simulink model "PMSM_FOC_sensorless"  (R2026a)
settings: Solver=FixedStepDiscrete  StopTime=10  FixedStep=Ts  EnableMultiTasking=on
InitFcn:
  | ParameterInit
undefined symbols (not defined in the file): drive, FAKF, motor, Ts
libraries: simulink x10, mcbhdlcontrolslib x10, matrix_library x8, mcbcontrolslib x6, mcbpositiondecoderlib x3, mcbsensorlessestimatorlib x2, mcbeeMathTransformLib x2, slpidlib x2, sl_discontinuities x1, mcbplantlib x1, autolibpmsminterior x1, realtime_pacer_lib x1
(part 2 of 3)

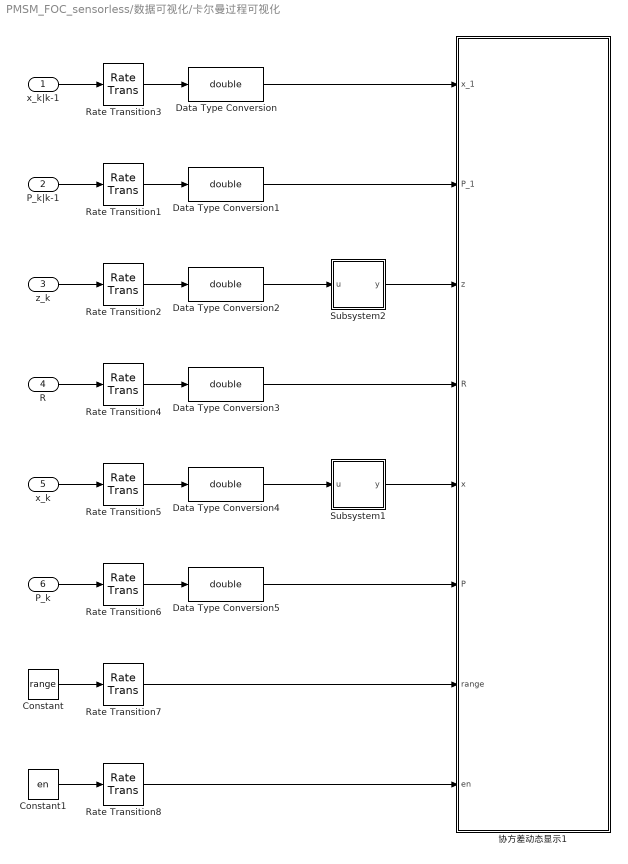
== system PMSM_FOC_sensorless/数据可视化/卡尔曼过程可视化 ==
  x_k|k-1 : Inport
  P_k|k-1 : Inport  Port=2
  z_k : Inport  Port=3
  R : Inport  Port=4
  x_k : Inport  Port=5
  P_k : Inport  Port=6
  Constant : Constant  Value=range
  Constant1 : Constant  Value=en
  Data Type Conversion{,1..5} (6 alike) : DataTypeConversion  OutDataTypeStr=double  SaturateOnIntegerOverflow=off  RndMeth=Floor
  Rate Transition{1..8} (8 alike) : RateTransition  OutPortSampleTime=1/plot_freq
  Subsystem1 : Subsystem
  Subsystem2 : Subsystem
  协方差动态显示1 : MATLAB Function  TreatAsAtomicUnit=on
  wires:
  z_k/1 -> Rate Transition2/1
  x_k/1 -> Rate Transition5/1
  R/1 -> Rate Transition4/1
  Rate Transition2/1 -> Data Type Conversion2/1
  P_k|k-1/1 -> Rate Transition1/1
  x_k|k-1/1 -> Rate Transition3/1
  Rate Transition5/1 -> Data Type Conversion4/1
  Rate Transition4/1 -> Data Type Conversion3/1
  P_k/1 -> Rate Transition6/1
  Rate Transition1/1 -> Data Type Conversion1/1
  Rate Transition3/1 -> Data Type Conversion/1
  Data Type Conversion4/1 -> Subsystem1/1(u)
  Data Type Conversion2/1 -> Subsystem2/1(u)
  Data Type Conversion/1 -> 协方差动态显示1/1(x_1)
  Data Type Conversion3/1 -> 协方差动态显示1/4(R)
  Subsystem2/1(y) -> 协方差动态显示1/3(z)
  Data Type Conversion1/1 -> 协方差动态显示1/2(P_1)
  Subsystem1/1(y) -> 协方差动态显示1/5(x)
  Data Type Conversion5/1 -> 协方差动态显示1/6(P)
  Constant/1 -> Rate Transition7/1
  Rate Transition6/1 -> Data Type Conversion5/1
  Constant1/1 -> Rate Transition8/1
  Rate Transition7/1 -> 协方差动态显示1/7(range)
  Rate Transition8/1 -> 协方差动态显示1/8(en)

== system PMSM_FOC_sensorless/Encoder&Hall/霍尔传感器/Subsystem ==
  MtrPos : Inport
  Constant6 : Constant  Value=pi/6  OutDataTypeStr=single
  Constant7 : Constant  Value=6  OutDataTypeStr=int16
  Data Type Conversion : DataTypeConversion  OutDataTypeStr=single  SaturateOnIntegerOverflow=off  RndMeth=Floor
  Data Type Conversion1 : DataTypeConversion  OutDataTypeStr=int16  SaturateOnIntegerOverflow=off  RndMeth=Floor
  Gain : Gain  Gain=6/(2*pi)
  Mechanical to Electrical Position : mcbpositiondecoderlib/Mechanical to Electrical Position  PolePairsInputType=Specify via dialog  NrPP=motor.P  selectedRange=Radians  MechOfstInputType=Specify via dialog  mechOffsetIn=0  maxAngleIn=2*pi  InputDataType=single  VariantSelect=floating-point
  Mod : Math  Operator=mod
  Sum : Sum  Inputs=|++
  Phase : Outport
  wires:
  Mod/1 -> Phase/1
  Data Type Conversion1/1 -> Mod/1
  Gain/1 -> Data Type Conversion1/1
  Sum/1 -> Gain/1
  Constant6/1 -> Sum/2
  Constant7/1 -> Mod/2
  Data Type Conversion/1 -> Mechanical to Electrical Position/1  "ElecAngle"
  MtrPos/1 -> Data Type Conversion/1
  Mechanical to Electrical Position/1 -> Sum/1

== system PMSM_FOC_sensorless/FOC/Observer/AKF ==
  u_k : Inport
  z_k : Inport  Port=2
  协方差估计 : Subsystem
  协方差计算 : Subsystem
  状态观测 : Subsystem
  x_k : Outport
  tag scope: K=global, Q=global, R=global, S=global, T=global
  wires:
  协方差估计/1(R) -> 协方差计算/1(R), [R]  "R"
  u_k/1 -> 状态观测/1(u)
  z_k/1 -> 状态观测/2(z)
  状态观测/1(x^) -> x_k/1  "x^"
  状态观测/3(e^) -> 协方差估计/2(e^)  "e^"
  状态观测/2(e~) -> 协方差估计/1(e~)  "e~"
  协方差计算/2(S) -> [S], 协方差估计/3(S)  "S"
  协方差估计/2(Q) -> [Q], 协方差计算/2(Q)  "Q"
  协方差计算/1(K) -> [K], 状态观测/3(K)  "K"
  协方差计算/3(T) -> [T], 协方差估计/4(T)  "T"

== system PMSM_FOC_sensorless/FOC/Observer/位置提取 ==
  Eαβ : Inport
  θ_sincos : Inport  Port=2
  Constant : Constant  Value=motor.psi  OutDataTypeStr=single
  Demux : Demux  Outputs=2
  Divide3 : Product  Inputs=/*
  Gain : Gain  Gain=[-1 1]  Multiplication=Matrix(K*u)
  Gain1 : Gain  Gain=motor.P
  Gain2 : Gain  Gain=-1
  Mux : Mux  Inputs=2
  Product : Product
  Product1 : Product
  Sign : Signum
  Unit Delay : UnitDelay  SampleTime=-1
  幅角 : mcbcontrolslib/atan2  ApproximationMethod=None  NumberOfIterations=11  NumberOfDataPoints=16  InterpMethod=Flat  outputUnit=Radians  TableDataTypeStr=Inherit: Inherit via input
  ωθ : Outport
  wires:
  Constant/1 -> Gain1/1
  Gain1/1 -> Divide3/1
  幅角/1 -> Mux/2
  θ_sincos/1 -> Unit Delay/1
  Unit Delay/1 -> Product/1
  Product/1 -> Gain/1
  Gain/1 -> Divide3/2, Sign/1
  Divide3/1 -> Mux/1
  Mux/1 -> ωθ/1
  Demux/2 -> 幅角/2
  Demux/1 -> Gain2/1
  Gain2/1 -> 幅角/1
  Eαβ/1 -> Product/2, Product1/2
  Sign/1 -> Product1/1
  Product1/1 -> Demux/1

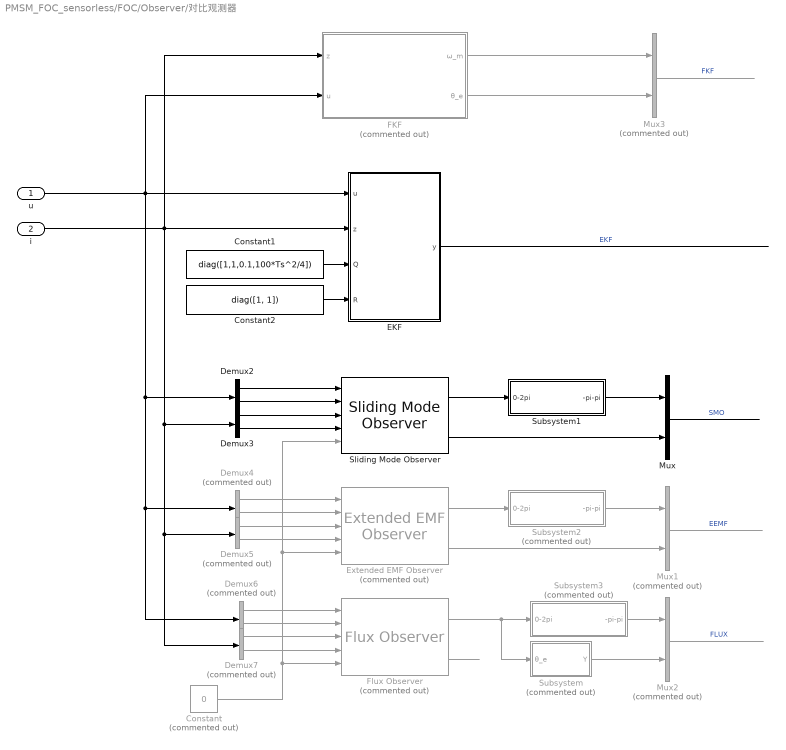
== system PMSM_FOC_sensorless/FOC/Observer/对比观测器 ==
  u : Inport
  i : Inport  Port=2
  Constant : Constant  Commented=on  Value=0  OutDataTypeStr=single
  Constant1 : Constant  Value=diag([1,1,0.1,100*Ts^2/4])  OutDataTypeStr=single
  Constant2 : Constant  Value=diag([1, 1])  OutDataTypeStr=single
  Demux2 : Demux  Outputs=2
  Demux3 : Demux  Outputs=2
  Demux{4..7} (4 alike) : Demux  Commented=on  Outputs=2
  EKF : Subsystem
  Extended EMF Observer : mcbsensorlessestimatorlib/Extended EMF Observer  Commented=on  InputUnit=SI unit  PosOut=Electrical position  BlkSampleTime=Ts  StatorResistance=motor.Rs  StatorDaxisInductance=motor.Ls  StatorQaxisInductance=motor.Ls  MaxApplicationSpeed=3000  PolePairs=motor.P  MaxStatorVoltage=12*sqrt(3)  MaxStatorCurrent=10  Alpha=50  EEMFCutoffFreq=50  Kp=250  Ki=200000  N_points=1024  SpeedCutoffFreq=50  PositionUnit=Radians  PositionDataType=single  SpeedUnit=Radians/sec  PerUnitSpeed=6000  SpeedDataType=single  TableDatatype=single
      settings: LibrarySourceBlock=mcblib/Sensorless Estimators/Extended EMF Observer
  FKF : Subsystem  Commented=on
  Flux Observer : mcbpositiondecoderlib/Flux Observer  Commented=on  MotorSelection=PMSM  DataTypeSelect=off  BlockInputUnit=Per-unit  PerUnitVoltage=12*sqrt(3)  PerUnitCurrent=10  PositionSelect=on  FluxSelect=off  TorqueSelect=on  PolePairs=4  StatorResistance=0.36  StatorDAxisInductance=0.2e-3  StatorLeakageInductance=0.0068  RotorLeakageInductance=0.0068  MagnetizingInductance=0.0300  CutoffFreq=50  BlockSampleTime=Ts  ParameterBusInput=off  PositionUnit=Radians  PositionDatatype=single  FluxUnit=Weber  PerUnitFlux=0.1  FluxDatatype=single  TorqueUnit=Nm  PerUnitTorque=100  TorqueDatatype=single  DataType=0
      settings: LibrarySourceBlock=mcblib/Sensorless Estimators/Flux Observer
  Mux : Mux  Inputs=2
  Mux1 : Mux  Commented=on  Inputs=2
  Mux2 : Mux  Commented=on  Inputs=2
  Mux3 : Mux  Commented=on  Inputs=2
  Sliding Mode Observer : mcbsensorlessestimatorlib/Sliding Mode Observer  InputUnit=Per-unit  BlkSampleTime=Ts  StatorResistance=motor.Rs  StatorInductance=motor.Ls  MaxApplicationSpeed=3000  PolePairs=motor.P  MaxStatorVoltage=12*sqrt(3)  MaxStatorCurrent=10  DisturbanceObserverGain=0.9  CurrentObserverGain=0.5  CutoffFreq=600  PositionUnit=Radians  PositionDataType=single  SpeedUnit=Radians/sec  PerUnitSpeed=6000  SpeedDataType=single
      settings: LibrarySourceBlock=mcblib/Sensorless Estimators/Sliding Mode Observer
  Subsystem : Subsystem  Commented=on
  Subsystem1 : Subsystem
  Subsystem2 : Subsystem  Commented=on
  Subsystem3 : Subsystem  Commented=on
  wires:
  Demux3/2 -> Sliding Mode Observer/4
  Demux2/2 -> Sliding Mode Observer/2
  Demux2/1 -> Sliding Mode Observer/1
  Flux Observer/2 -> ?
  Sliding Mode Observer/2 -> Mux/2
  Demux3/1 -> Sliding Mode Observer/3
  Demux6/2 -> Flux Observer/2
  Demux7/1 -> Flux Observer/3
  Demux6/1 -> Flux Observer/1
  Demux7/2 -> Flux Observer/4
  Constant/1 -> Flux Observer/5, Extended EMF Observer/5, Sliding Mode Observer/5
  Flux Observer/1 -> Subsystem/1(θ_e), Subsystem3/1(0-2pi)
  Extended EMF Observer/1 -> Subsystem2/1(0-2pi)
  Sliding Mode Observer/1 -> Subsystem1/1(0-2pi)
  Extended EMF Observer/2 -> Mux1/2
  Demux5/2 -> Extended EMF Observer/4
  Demux5/1 -> Extended EMF Observer/3
  Demux4/1 -> Extended EMF Observer/1
  Demux4/2 -> Extended EMF Observer/2
  u/1 -> EKF/1(u), FKF/2(u), Demux2/1, Demux4/1, Demux6/1
  Constant2/1 -> EKF/4(R)
  Constant1/1 -> EKF/3(Q)
  i/1 -> Demux3/1, Demux5/1, Demux7/1, FKF/1(z), EKF/2(z)
  EKF/1(y) -> ?  "EKF"
  Subsystem/1(Y) -> Mux2/2
  Mux/1 -> ?  "SMO"
  Mux1/1 -> ?  "EEMF"
  Mux2/1 -> ?  "FLUX"
  FKF/1(ω_m) -> Mux3/1
  FKF/2(θ_e) -> Mux3/2
  Mux3/1 -> ?  "FKF"
  Subsystem1/1(-pi-pi) -> Mux/1
  Subsystem2/1(-pi-pi) -> Mux1/1
  Subsystem3/1(-pi-pi) -> Mux2/1

== system PMSM_FOC_sensorless/FOC/Observer/角度转换 ==
  θ : Inport
  Mux1 : Mux  Inputs=2
  SinCos : Trigonometry  Operator=sincos
  sincos : Outport
  wires:
  SinCos/1 -> Mux1/1
  θ/1 -> SinCos/1
  SinCos/2 -> Mux1/2
  Mux1/1 -> sincos/1

== system PMSM_FOC_sensorless/FOC/Observer/计算转子反电动势 ==
  Iαβ : Inport
  Uαβ : Inport  Port=2
  Sum5 : Sum  Inputs=+--
  滞后补偿 : DiscreteFilter  Numerator=[0 0 1 1]  Denominator=[2 0 0 0]
  电感分压 : simulink/Discrete/Discrete Derivative  gainval=motor.Ls  ICPrevScaledInput=0.0  OutMin=[]  OutMax=[]  OutDataType=fixdt(1, 16)  OutScaling=2^-10  DoSatur=off
  电阻分压 : Gain  Gain=motor.Rs
  Eαβ : Outport
  tag scope: E_alphabeta=global
  wires:
  电感分压/1 -> Sum5/3
  电阻分压/1 -> Sum5/2
  Uαβ/1 -> 滞后补偿/1
  Iαβ/1 -> 电感分压/1, 电阻分压/1
  滞后补偿/1 -> Sum5/1
  Sum5/1 -> Eαβ/1, [E_alphabeta]

== system PMSM_FOC_sensorless/FOC/Observer/转矩计算 ==
  θ_sincos : Inport
  I_αβ : Inport  Port=2
  Constant : Constant  Value=motor.psi  OutDataTypeStr=single
  Divide1 : Product  Inputs=**
  Gain : Gain  Gain=[-1 1]  Multiplication=Matrix(K*u)
  Gain1 : Gain  Gain=motor.P
  Gain2 : Gain  Gain=1.5
  Product3 : Product
  Unit Delay : UnitDelay  SampleTime=-1
  T : Outport
  wires:
  Product3/1 -> Gain/1
  Constant/1 -> Gain1/1
  Divide1/1 -> Gain2/1
  Gain/1 -> Divide1/1
  Unit Delay/1 -> Product3/1
  I_αβ/1 -> Product3/2
  θ_sincos/1 -> Unit Delay/1
  Gain1/1 -> Divide1/2
  Gain2/1 -> T/1

== system PMSM_FOC_sensorless/FOC/PWM调制&故障诊断/故障诊断 ==
  note: 过流保护
  note: 故障码位数说明（暂定）
      |
      | 位
      | 15
      | 14
      | 13
      | 12
      | 11
      | 10
      | 9
      | 8
      | 7
      | 6
      | 5
      | 4
      | 3
      | 2
      | 1
      | 0
      |
      | 说明
      | -
      | -
      | -
      | -
      | -
      | -
      | -
      | -
      | -
      | -
      | -
      | -
      | 过热
      | 过压
      | 欠压
      | 过流
      |
      | 位
      | 31
      | 30
      | 29
      | 28
      | 27
      | 26
      | 25
      | 24
      | 23
      | 22
      | 21
      | 20
      | 19
      | 18
      | 17
      | 16
      |
      | 说明
      | ​
      | ​
      | ​
      | ​
      | ​
      | ​
      | ​
      | ​
      | ​
      | ​
      | ​
      | ​
      | ​
      | ​
      | ​
      | ​
  note: 欠压过压保护
  I_abc : Inport
  U_bus : Inport  Port=2
  Abs : Abs  SaturateOnIntegerOverflow=off
  Bitwise Operator1 : simulink/Logic and Bit Operations/Bitwise Operator  logicop=OR  UseBitMask=off  NumInputPorts=3  BitMask=bin2dec('11011001')  BitMaskRealWorld=Stored Integer
  Constant1 : Constant  Value=drive.V_min
  Constant2 : Constant  Value=drive.I_max
  Constant3 : Constant  Value=drive.V_max
  Gain1 : Gain  Gain=0x2  OutDataTypeStr=uint32
  Gain2 : Gain  Gain=0x4  OutDataTypeStr=uint32
  Gain4 : Gain  Gain=0x1  OutDataTypeStr=uint32
  IIR Filter : mcbhdlcontrolslib/IIR Filter  VariantControl=Low Pass Filter  VariantSelect=Low-pass  FilterConstantInputType=Specify via dialog  Filter_constant=0.1  advancedSettings=off  Ts=50e-6  cutOff_freq=353.6777
  Max : MinMax  Function=max
  OR : Logic  Operator=OR  IconShape=distinctive  AllPortsSameDT=off  OutDataTypeStr=boolean
  Relational Operator : RelationalOperator  Operator=>  OutDataTypeStr=boolean  RndMeth=Simplest  InputSameDT=off
  Relational Operator1 : RelationalOperator  Operator=>  OutDataTypeStr=boolean  RndMeth=Simplest  InputSameDT=off
  Relational Operator2 : RelationalOperator  Operator=<  OutDataTypeStr=boolean  RndMeth=Simplest  InputSameDT=off
  Unit Delay : UnitDelay  SampleTime=-1
  Err_code : Outport
  tag scope: Err_code=global
  wires:
  U_bus/1 -> Relational Operator1/1, Relational Operator2/1
  I_abc/1 -> IIR Filter/1
  Abs/1 -> Max/1
  Constant2/1 -> Relational Operator/2
  Constant1/1 -> Relational Operator2/2
  Relational Operator2/1 -> Gain1/1
  Max/1 -> Relational Operator/1
  Relational Operator1/1 -> Gain2/1
  Constant3/1 -> Relational Operator1/2
  Unit Delay/1 -> OR/1
  Bitwise Operator1/1 -> [Err_code], Err_code/1
  IIR Filter/1 -> Abs/1
  Relational Operator/1 -> OR/2
  Gain2/1 -> Bitwise Operator1/3
  Gain1/1 -> Bitwise Operator1/2
  Gain4/1 -> Bitwise Operator1/1
  OR/1 -> Unit Delay/1, Gain4/1

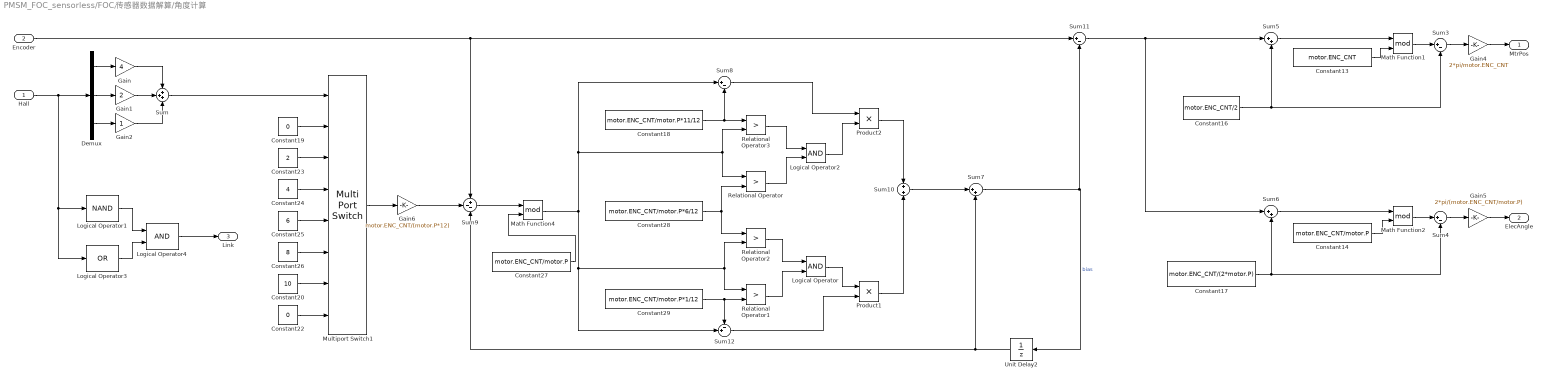
== system PMSM_FOC_sensorless/FOC/传感器数据解算/角度计算 ==
  Hall : Inport
  Encoder : Inport  Port=2
  Constant13 : Constant  Value=motor.ENC_CNT  OutDataTypeStr=int16
  Constant14 : Constant  Value=motor.ENC_CNT/motor.P  OutDataTypeStr=int16
  Constant16 : Constant  Value=motor.ENC_CNT/2  OutDataTypeStr=int16
  Constant17 : Constant  Value=motor.ENC_CNT/(2*motor.P)  OutDataTypeStr=int16
  Constant18 : Constant  Value=motor.ENC_CNT/motor.P*11/12  OutDataTypeStr=int16
  Constant19 : Constant  Value=0  OutDataTypeStr=int16
  Constant20 : Constant  Value=10  OutDataTypeStr=int16
  Constant22 : Constant  Value=0  OutDataTypeStr=int16
  Constant23 : Constant  Value=2  OutDataTypeStr=int16
  Constant24 : Constant  Value=4  OutDataTypeStr=int16
  Constant25 : Constant  Value=6  OutDataTypeStr=int16
  Constant26 : Constant  Value=8  OutDataTypeStr=int16
  Constant27 : Constant  Value=motor.ENC_CNT/motor.P  OutDataTypeStr=int16
  Constant28 : Constant  Value=motor.ENC_CNT/motor.P*6/12  OutDataTypeStr=int16
  Constant29 : Constant  Value=motor.ENC_CNT/motor.P*1/12  OutDataTypeStr=int16
  Demux : Demux  Outputs=3
  Gain : Gain  Gain=4
  Gain1 : Gain  Gain=2
  Gain2 : Gain
  Gain4 : Gain  Gain=2*pi/motor.ENC_CNT  OutDataTypeStr=single
  Gain5 : Gain  Gain=2*pi/(motor.ENC_CNT/motor.P)  OutDataTypeStr=single
  Gain6 : Gain  Gain=motor.ENC_CNT/(motor.P*12)  OutDataTypeStr=int16
  Logical Operator : Logic  AllPortsSameDT=off  OutDataTypeStr=boolean
  Logical Operator1 : Logic  Operator=NAND  Inputs=1  IconShape=distinctive  AllPortsSameDT=off  OutDataTypeStr=boolean
  Logical Operator2 : Logic  AllPortsSameDT=off  OutDataTypeStr=boolean
  Logical Operator3 : Logic  Operator=OR  Inputs=1  IconShape=distinctive  AllPortsSameDT=off  OutDataTypeStr=boolean
  Logical Operator4 : Logic  IconShape=distinctive  AllPortsSameDT=off  OutDataTypeStr=boolean
  Math Function1 : Math  Operator=mod
  Math Function2 : Math  Operator=mod
  Math Function4 : Math  Operator=mod
  Multiport Switch1 : MultiPortSwitch  DataPortOrder=Specify indices  DataPortIndices={5,4,6,2,3,1}  DataPortForDefault=Additional data port  DiagnosticForDefault=None  SaturateOnIntegerOverflow=off  InputSameDT=off
  Product1 : Product  Inputs=**
  Product2 : Product  Inputs=**
  Relational Operator{,1..3} (4 alike) : RelationalOperator  Operator=>  OutDataTypeStr=boolean  RndMeth=Simplest  InputSameDT=off
  Sum : Sum  Inputs=+++
  Sum10 : Sum  Inputs=+|+
  Sum{3..4,8,11} (4 alike) : Sum  Inputs=|+-
  Sum12 : Sum  Inputs=-+|
  Sum5 : Sum  Inputs=|++
  Sum6 : Sum  Inputs=|++
  Sum7 : Sum  Inputs=|++
  Sum9 : Sum  Inputs=+--
  Unit Delay2 : UnitDelay  SampleTime=-1
  MtrPos : Outport
  ElecAngle : Outport  Port=2
  Link : Outport  Port=3
  wires:
  Sum6/1 -> Math Function2/1
  Sum5/1 -> Math Function1/1
  Constant17/1 -> Sum6/2, Sum4/2
  Constant16/1 -> Sum3/2, Sum5/2
  Math Function2/1 -> Sum4/1
  Math Function1/1 -> Sum3/1
  Gain5/1 -> ElecAngle/1
  Gain4/1 -> MtrPos/1
  Sum3/1 -> Gain4/1
  Constant14/1 -> Math Function2/2
  Sum11/1 -> Sum6/1, Sum5/1
  Constant13/1 -> Math Function1/2
  Sum4/1 -> Gain5/1
  Demux/1 -> Gain/1
  Hall/1 -> Demux/1, Logical Operator3/1, Logical Operator1/1
  Gain/1 -> Sum/1
  Demux/2 -> Gain1/1
  Demux/3 -> Gain2/1
  Gain1/1 -> Sum/2
  Gain2/1 -> Sum/3
  Logical Operator4/1 -> Link/1
  Logical Operator1/1 -> Logical Operator4/1
  Logical Operator3/1 -> Logical Operator4/2
  Constant26/1 -> Multiport Switch1/6
  Constant24/1 -> Multiport Switch1/4
  Constant25/1 -> Multiport Switch1/5
  Constant20/1 -> Multiport Switch1/7
  Relational Operator2/1 -> Logical Operator/1
  Constant28/1 -> Relational Operator/2, Relational Operator2/1
  Constant27/1 -> Math Function4/2
  Relational Operator/1 -> Logical Operator2/2
  Constant19/1 -> Multiport Switch1/2
  Unit Delay2/1 -> Sum7/2, Sum9/3
  Sum9/1 -> Math Function4/1
  Constant22/1 -> Multiport Switch1/8
  Logical Operator/1 -> Product1/1
  Multiport Switch1/1 -> Gain6/1
  Constant29/1 -> Sum12/1, Relational Operator1/2
  Product1/1 -> Sum10/2
  Relational Operator3/1 -> Logical Operator2/1
  Constant18/1 -> Sum8/2, Relational Operator3/1
  Sum8/1 -> Product2/1
  Math Function4/1 -> Sum8/1, Relational Operator/1, Relational Operator3/2, Sum12/2, Relational Operator2/2, Relational Operator1/1
  Gain6/1 -> Sum9/2
  Sum12/1 -> Product1/2
  Constant23/1 -> Multiport Switch1/3
  Sum7/1 -> Unit Delay2/1, Sum11/2  "bias"
  Relational Operator1/1 -> Logical Operator/2
  Encoder/1 -> Sum9/1, Sum11/1
  Logical Operator2/1 -> Product2/2
  Product2/1 -> Sum10/1
  Sum10/1 -> Sum7/1
  Sum/1 -> Multiport Switch1/1

== system PMSM_FOC_sensorless/FOC/传感器数据解算/转速计算 ==
  note: 五阶巴特沃斯滤波器
  Encoder : Inport
  Constant3 : Constant  Value=motor.ENC_CNT/2  OutDataTypeStr=int16
  Constant4 : Constant  Value=-motor.ENC_CNT/2  OutDataTypeStr=int16
  Difference : simulink/Discrete/Difference  ICPrevInput=0.0  OutMin=[]  OutMax=[]  OutDataType=fixdt(1, 16)  OutScaling=2^-10  DoSatur=off
  Gain : Gain  Gain=2*pi/motor.ENC_CNT  OutDataTypeStr=single
  Gain1 : Gain  Gain=-motor.ENC_CNT  OutDataTypeStr=int16
  Gain2 : Gain  Gain=motor.ENC_CNT  OutDataTypeStr=int16
  Gain3 : Gain  Gain=1/Ts  OutDataTypeStr=single
  IIR Filter{,1..4} (5 alike) : mcbhdlcontrolslib/IIR Filter  VariantControl=Low Pass Filter  VariantSelect=Low-pass  FilterConstantInputType=Specify via dialog  Filter_constant=0.5  advancedSettings=off  Ts=50e-6  cutOff_freq=3183.0989
  Relational Operator : RelationalOperator  Operator=<  RndMeth=Simplest  InputSameDT=off
  Relational Operator1 : RelationalOperator  Operator=<  RndMeth=Simplest  InputSameDT=off
  Sum2 : Sum  Inputs=+++
  MtrSpeed : Outport
  wires:
  Difference/1 -> Relational Operator1/2, Relational Operator/1, Sum2/2
  Gain2/1 -> Sum2/3
  Gain/1 -> IIR Filter/1
  Constant3/1 -> Relational Operator1/1
  Gain3/1 -> Gain/1
  Gain1/1 -> Sum2/1
  Constant4/1 -> Relational Operator/2
  Relational Operator1/1 -> Gain1/1
  Encoder/1 -> Difference/1
  Relational Operator/1 -> Gain2/1
  IIR Filter/1 -> IIR Filter1/1
  IIR Filter1/1 -> IIR Filter2/1
  Sum2/1 -> Gain3/1
  IIR Filter2/1 -> IIR Filter3/1
  IIR Filter3/1 -> IIR Filter4/1
  IIR Filter4/1 -> MtrSpeed/1

== system PMSM_FOC_sensorless/FOC/全速域电流分配/MJPA ==
  note: $J\left( u_{bus},\omega _m,i_d \right) =-L\frac{{\omega _{mc}}^2}{{\omega _{mc}}^2+{\omega _m}^2}i_d+{Mi_d}^2+\frac{N}{{u_{bus}}^2/3-p_n\omega _m\left( \psi _f+L_di_d \right) ^2}$
  Vbus : Inport
  ω_m : Inport  Port=2
  IIR Filter : mcbhdlcontrolslib/IIR Filter  VariantControl=Low Pass Filter  VariantSelect=Low-pass  FilterConstantInputType=Specify via dialog  Filter_constant=0.1  advancedSettings=off  Ts=50e-6  cutOff_freq=353.6777
  J_function1 : Subsystem  ReferencedSubsystem=J_function
  J_function2 : Subsystem  Commented=on  ReferencedSubsystem=J_function
  J_function3 : Subsystem  ReferencedSubsystem=J_function
  Saturation1 : Saturate  UpperLimit=0.1  LowerLimit=-0.1
  Saturation2 : Saturate  UpperLimit=min(motor.I_rated*1.2)  LowerLimit=max(-motor.I_rated*1.2, -motor.psi/motor.Ls)
  Subsystem2 : Subsystem  Commented=on
  Sum2 : Sum  Inputs=|++
  Sum3 : Sum  Inputs=+|-
  Sum4 : Sum  Inputs=|-+
  Unit Delay : UnitDelay  SampleTime=-1
  Δid : Constant  Value=1e-2  OutDataTypeStr=single
  收敛系数 : Gain  Gain=100
  i*_d : Outport
  wires:
  Saturation1/1 -> Sum4/1
  Δid/1 -> Sum2/1
  Sum2/1 -> J_function1/1
  J_function1/1 -> Sum3/1
  Sum3/1 -> 收敛系数/1  "ΔJ"
  Unit Delay/1 -> Sum4/2, Sum2/2, J_function3/1
  J_function3/1 -> Sum3/2
  Vbus/1 -> J_function3/3, J_function1/3
  收敛系数/1 -> Saturation1/1
  ω_m/1 -> J_function3/2, J_function1/2
  Sum4/1 -> Saturation2/1  "i_d"
  Saturation2/1 -> IIR Filter/1, Unit Delay/1
  IIR Filter/1 -> i*_d/1

== system PMSM_FOC_sensorless/FOC/坐标变换/Subsystem11 ==
  angle : Inport
  Mux : Mux  Inputs=2
  SinCos : Trigonometry  Operator=sincos
  sincos : Outport
  wires:
  SinCos/1 -> Mux/1
  Mux/1 -> sincos/1
  SinCos/2 -> Mux/2
  angle/1 -> SinCos/1

== system PMSM_FOC_sensorless/FOC/坐标变换/Subsystem2 ==
  αβ : Inport
  sincos : Inport  Port=2
  Demux : Demux  Outputs=2
  Demux1 : Demux  Outputs=2
  Mux : Mux  Inputs=2
  Park Transform : mcbeeMathTransformLib/Clarke to Park Angle Transform  AxisAlignment=D-axis  UseWithEmbedded=on  PhaseInput=Two inputs  ThetaInput=Sine and Cosine electrical position  AngleInput=Per-unit  N_points=1024
  dq : Outport
  wires:
  sincos/1 -> Demux1/1
  Demux/2 -> Park Transform/2
  Mux/1 -> dq/1
  Demux/1 -> Park Transform/1
  Demux1/1 -> Park Transform/3
  αβ/1 -> Demux/1
  Demux1/2 -> Park Transform/4
  Park Transform/1 -> Mux/1
  Park Transform/2 -> Mux/2

== system PMSM_FOC_sensorless/FOC/坐标变换/Subsystem3 ==
  abc : Inport
  Gain : Gain  Gain=[2/3 -1/3 -1/3;0 sqrt(3)/3 -sqrt(3)/3]  Multiplication=Matrix(K*u)
  αβ : Outport
  wires:
  abc/1 -> Gain/1
  Gain/1 -> αβ/1

== system PMSM_FOC_sensorless/FOC/坐标变换/Subsystem4 ==
  αβ : Inport
  Demux1 : Demux  Outputs=2
  Gain : Gain  Gain=sqrt(3)/2
  Mux1 : Mux  Inputs=3
  PWM Reference Generator : mcbcontrolslib/PWM Reference Generator  modType=SVM: space vector modulation  inSignal=Valphabeta  expandVoltageInput=on  inputUnits=Per-unit  LimitModulation=off  enableVoltage=on  enableModulationSignal=off  enableDutyCycle=off  expandVoltageOutput=on
  abc : Outport
  wires:
  αβ/1 -> Demux1/1
  Mux1/1 -> Gain/1
  Demux1/1 -> PWM Reference Generator/1
  Demux1/2 -> PWM Reference Generator/2
  PWM Reference Generator/3 -> Mux1/3
  PWM Reference Generator/1 -> Mux1/1
  PWM Reference Generator/2 -> Mux1/2
  Gain/1 -> abc/1

== system PMSM_FOC_sensorless/FOC/坐标变换/Subsystem5 ==
  dq : Inport
  sincos : Inport  Port=2
  Demux : Demux  Outputs=2
  Demux1 : Demux  Outputs=2
  Inverse Park Transform : mcbeeMathTransformLib/Park to Clarke Angle Transform  AxisAlignment=D-axis  UseWithEmbedded=on  PhaseInput=Two inputs  ThetaInput=Sine and Cosine electrical position  AngleInput=Per-unit  N_points=1024
  Mux : Mux  Inputs=2
  αβ : Outport
  wires:
  sincos/1 -> Demux1/1
  Demux1/1 -> Inverse Park Transform/3
  Demux/1 -> Inverse Park Transform/1
  dq/1 -> Demux/1
  Demux/2 -> Inverse Park Transform/2
  Inverse Park Transform/1 -> Mux/1
  Inverse Park Transform/2 -> Mux/2
  Mux/1 -> αβ/1
  Demux1/2 -> Inverse Park Transform/4

== system PMSM_FOC_sensorless/FOC/电流控制/前馈控制1 ==
  ω : Inport
  IdqRef : Inport  Port=2
  IdqFb : Inport  Port=3
  Demux : Demux  Outputs=2
  Demux1 : Demux  Outputs=2
  Discrete Derivative : simulink/Discrete/Discrete Derivative  gainval=motor.Ls  ICPrevScaledInput=0.0  OutMin=[]  OutMax=[]  OutDataType=fixdt(1, 16)  OutScaling=2^-10  DoSatur=off
  Discrete Derivative1 : simulink/Discrete/Discrete Derivative  gainval=motor.Ls  ICPrevScaledInput=0.0  OutMin=[]  OutMax=[]  OutDataType=fixdt(1, 16)  OutScaling=2^-10  DoSatur=off
  Divide1 : Product  Inputs=**
  Divide2 : Product  Inputs=**
  Ld : Gain  Gain=motor.P*motor.Ls
  Lq : Gain  Gain=motor.P*motor.Ls
  Mux : Mux  Inputs=2
  R1 : Gain  Gain=motor.Rs
  R2 : Gain  Gain=motor.Rs
  Sum : Sum  Inputs=+++
  Sum3 : Sum  Inputs=|++
  Sum4 : Sum  Inputs=++-
  转子磁链1 : Constant  Value=motor.P*motor.psi  VectorParams1D=off  OutDataTypeStr=single
  FeedForward : Outport
  wires:
  Demux1/1 -> Discrete Derivative/1  "id"
  Mux/1 -> FeedForward/1
  Discrete Derivative/1 -> Sum4/1
  Discrete Derivative1/1 -> Sum/1
  R1/1 -> Sum4/2  "电阻压降"
  R2/1 -> Sum/2  "电阻压降"
  Demux1/2 -> Discrete Derivative1/1  "iq"
  IdqRef/1 -> Demux1/1
  Sum4/1 -> Mux/1
  Sum/1 -> Mux/2
  Divide1/1 -> Sum/3
  Divide2/1 -> Sum4/3
  IdqFb/1 -> Demux/1
  Demux/2 -> R2/1, Lq/1  "iq*"
  Demux/1 -> Ld/1, R1/1  "id*"
  ω/1 -> Divide1/2, Divide2/2
  Sum3/1 -> Divide1/1
  Lq/1 -> Divide2/1  "定子磁链"
  转子磁链1/1 -> Sum3/2
  Ld/1 -> Sum3/1  "定子磁链"

== system PMSM_FOC_sensorless/FOC/电流控制/电压限幅 ==
  dq_in : Inport
  Limit : Inport  Port=2
  Divide1 : Product  Inputs=*/*
  Math Function1 : Math  Operator=square
  Relational Operator : RelationalOperator  Operator=>  OutDataTypeStr=boolean  RndMeth=Simplest  InputSameDT=off
  Sqrt : Sqrt
  Sum of Elements1 : Sum  Inputs=+
  Switch : Switch  Criteria=u2 > Threshold  SaturateOnIntegerOverflow=off  InputSameDT=off
  dq_out : Outport
  wires:
  dq_in/1 -> Math Function1/1, Switch/3, Divide1/3
  Limit/1 -> Divide1/1, Relational Operator/2
  Sqrt/1 -> Divide1/2, Relational Operator/1
  Sum of Elements1/1 -> Sqrt/1
  Switch/1 -> dq_out/1
  Math Function1/1 -> Sum of Elements1/1
  Relational Operator/1 -> Switch/2
  Divide1/1 -> Switch/1

== system PMSM_FOC_sensorless/FOC/电流控制/非线性补偿 ==
  U_dq : Inport
  Gain1 : Gain  Gain=[1/(motor.Rs+motor.Ls/Ts) 1/(motor.Rs+motor.Ls/Ts)]
  I_dq : Outport
  wires:
  Gain1/1 -> I_dq/1
  U_dq/1 -> Gain1/1

== system PMSM_FOC_sensorless/数据可视化/卡尔曼过程可视化/Subsystem1 ==
  u : Inport
  MATLAB Function : MATLAB Function  TreatAsAtomicUnit=on
  Unit Delay : UnitDelay  InitialCondition=zeros(2,buff_len)  SampleTime=-1
  y : Outport
  wires:
  MATLAB Function/1(y) -> y/1, Unit Delay/1
  Unit Delay/1 -> MATLAB Function/2(y_1)
  u/1 -> MATLAB Function/1(u)

== system PMSM_FOC_sensorless/数据可视化/卡尔曼过程可视化/Subsystem2 ==
  u : Inport
  MATLAB Function : MATLAB Function  TreatAsAtomicUnit=on
  Unit Delay : UnitDelay  InitialCondition=zeros(2,buff_len)  SampleTime=-1
  y : Outport
  wires:
  u/1 -> MATLAB Function/1(u)
  Unit Delay/1 -> MATLAB Function/2(y_1)
  MATLAB Function/1(y) -> Unit Delay/1, y/1

== system PMSM_FOC_sensorless/FOC/Observer/AKF/协方差估计 ==
  e~ : Inport
  e^ : Inport  Port=2
  S : Inport  Port=3
  T : Inport  Port=4
  Display : Display
  Display1 : Display
  Unit Delay1 : UnitDelay  InitialCondition=eye(2)  SampleTime=-1
  Unit Delay2 : UnitDelay  InitialCondition=eye(2)  SampleTime=-1
  乘法积分器 : Subsystem
  乘法积分器1 : Subsystem
  息差估计 : Subsystem
  残差估计 : Subsystem
  R : Outport
  Q : Outport  Port=2
  wires:
  e~/1 -> 息差估计/1(ωθ)
  残差估计/1(cov) -> 乘法积分器/1(S~)
  e^/1 -> 残差估计/1(ωθ)
  S/1 -> Unit Delay1/1
  息差估计/1(cov) -> 乘法积分器1/1(T~)
  Unit Delay1/1 -> 乘法积分器/2(S)
  乘法积分器1/1(R) -> Display1/1, R/1
  乘法积分器/1(Q) -> Display/1, Q/1
  T/1 -> Unit Delay2/1
  Unit Delay2/1 -> 乘法积分器1/2(T)

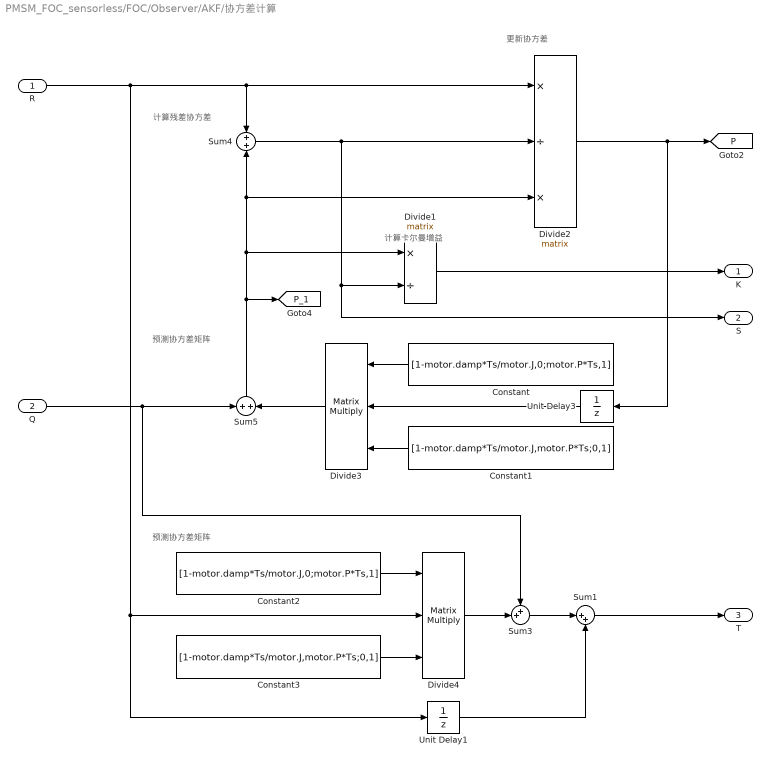
== system PMSM_FOC_sensorless/FOC/Observer/AKF/协方差计算 ==
  note: 预测协方差矩阵
  note: 计算残差协方差
  note: 计算卡尔曼增益
  note: 更新协方差
  note: 预测协方差矩阵
  R : Inport
  Q : Inport  Port=2
  Constant : Constant  Value=[1-motor.damp*Ts/motor.J,0;motor.P*Ts,1]  VectorParams1D=off  OutDataTypeStr=single
  Constant1 : Constant  Value=[1-motor.damp*Ts/motor.J,motor.P*Ts;0,1]  VectorParams1D=off  OutDataTypeStr=single
  Constant2 : Constant  Value=[1-motor.damp*Ts/motor.J,0;motor.P*Ts,1]  VectorParams1D=off  OutDataTypeStr=single
  Constant3 : Constant  Value=[1-motor.damp*Ts/motor.J,motor.P*Ts;0,1]  VectorParams1D=off  OutDataTypeStr=single
  Divide1 : Product  Inputs=*/  Multiplication=Matrix(*)
  Divide2 : Product  Inputs=*/*  Multiplication=Matrix(*)
  Divide3 : Product  Inputs=***  Multiplication=Matrix(*)
  Divide4 : Product  Inputs=***  Multiplication=Matrix(*)
  Sum1 : Sum  Inputs=|++
  Sum3 : Sum  Inputs=++|
  Sum4 : Sum  Inputs=+|+
  Sum5 : Sum  Inputs=+|+
  Unit Delay1 : UnitDelay  InitialCondition=eye(2)  SampleTime=-1
  Unit Delay3 : UnitDelay  InitialCondition=eye(2)  SampleTime=-1
  K : Outport
  S : Outport  Port=2
  T : Outport  Port=3
  tag scope: P=global, P_1=global
  wires:
  Sum5/1 -> [P_1], Divide1/1, Divide2/3, Sum4/2
  Constant/1 -> Divide3/1
  Divide2/1 -> [P], Unit Delay3/1
  Divide3/1 -> Sum5/2
  Constant1/1 -> Divide3/3
  Unit Delay3/1 -> Divide3/2
  Sum4/1 -> S/1, Divide1/2, Divide2/2
  Divide1/1 -> K/1
  Constant3/1 -> Divide4/3
  Constant2/1 -> Divide4/1
  Divide4/1 -> Sum3/2
  Sum3/1 -> Sum1/1
  R/1 -> Unit Delay1/1, Divide4/2, Divide2/1, Sum4/1
  Sum1/1 -> T/1
  Unit Delay1/1 -> Sum1/2
  Q/1 -> Sum3/1, Sum5/1

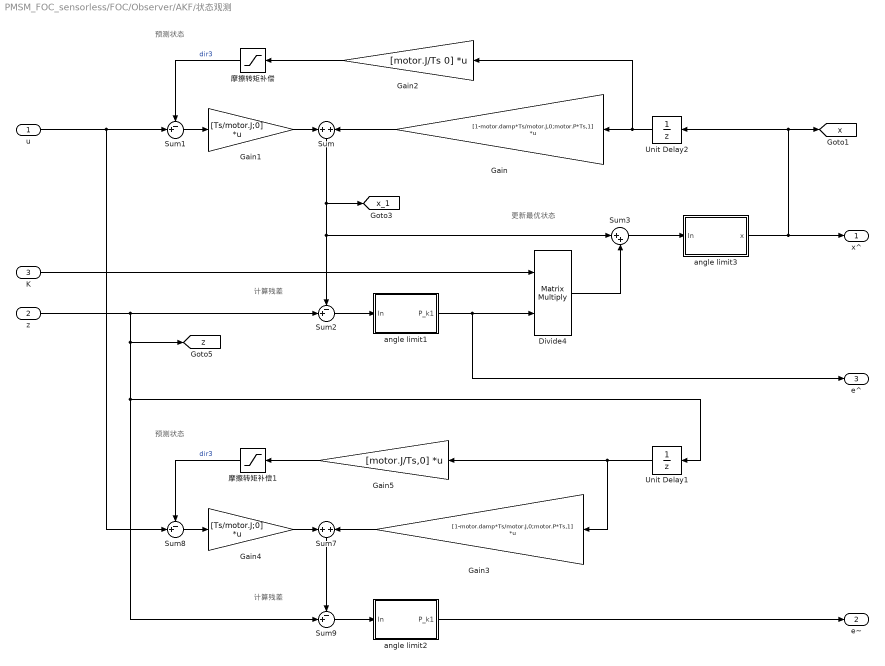
== system PMSM_FOC_sensorless/FOC/Observer/AKF/状态观测 ==
  note: 预测状态
  note: 计算残差
  note: 更新最优状态
  note: 预测状态
  note: 计算残差
  u : Inport
  z : Inport  Port=2
  K : Inport  Port=3
  Divide4 : Product  Inputs=**  Multiplication=Matrix(*)
  Gain : Gain  Gain=[1-motor.damp*Ts/motor.J,0;motor.P*Ts,1]  Multiplication=Matrix(K*u)
  Gain1 : Gain  Gain=[Ts/motor.J;0]  Multiplication=Matrix(K*u)
  Gain2 : Gain  Gain=[motor.J/Ts 0]  Multiplication=Matrix(K*u)
  Gain3 : Gain  Gain=[1-motor.damp*Ts/motor.J,0;motor.P*Ts,1]  Multiplication=Matrix(K*u)
  Gain4 : Gain  Gain=[Ts/motor.J;0]  Multiplication=Matrix(K*u)
  Gain5 : Gain  Gain=[motor.J/Ts,0]  Multiplication=Matrix(K*u)
  Sum : Sum  Inputs=+|+
  Sum{1..2,8..9} (4 alike) : Sum  Inputs=-+|
  Sum3 : Sum  Inputs=|++
  Sum7 : Sum  Inputs=+|+
  Unit Delay1 : UnitDelay  SampleTime=-1
  Unit Delay2 : UnitDelay  SampleTime=-1
  angle limit1 : Subsystem
  angle limit2 : Subsystem
  angle limit3 : Subsystem
  摩擦转矩补偿 : Saturate  UpperLimit=motor.fric  LowerLimit=-motor.fric
  摩擦转矩补偿1 : Saturate  UpperLimit=motor.fric  LowerLimit=-motor.fric
  x^ : Outport
  e~ : Outport  Port=2
  e^ : Outport  Port=3
  tag scope: x=global, x_1=global, z=global
  wires:
  Sum/1 -> [x_1], Sum2/1, Sum3/1
  angle limit1/1(P_k1) -> e^/1, Divide4/2
  Sum3/1 -> angle limit3/1(In)
  Gain4/1 -> Sum7/1
  Gain1/1 -> Sum/1
  Gain/1 -> Sum/2
  Gain3/1 -> Sum7/2
  Gain5/1 -> 摩擦转矩补偿1/1
  Unit Delay2/1 -> Gain2/1, Gain/1
  Divide4/1 -> Sum3/2
  Sum1/1 -> Gain1/1
  Gain2/1 -> 摩擦转矩补偿/1
  Sum7/1 -> Sum9/1
  angle limit3/1(x) -> x^/1, [x], Unit Delay2/1
  Sum9/1 -> angle limit2/1(In)
  Sum2/1 -> angle limit1/1(In)
  Sum8/1 -> Gain4/1
  Unit Delay1/1 -> Gain3/1, Gain5/1
  u/1 -> Sum1/2, Sum8/2
  z/1 -> Sum2/2, [z], Sum9/2, Unit Delay1/1
  K/1 -> Divide4/1
  angle limit2/1(P_k1) -> e~/1
  摩擦转矩补偿1/1 -> Sum8/1  "dir3"
  摩擦转矩补偿/1 -> Sum1/1  "dir3"

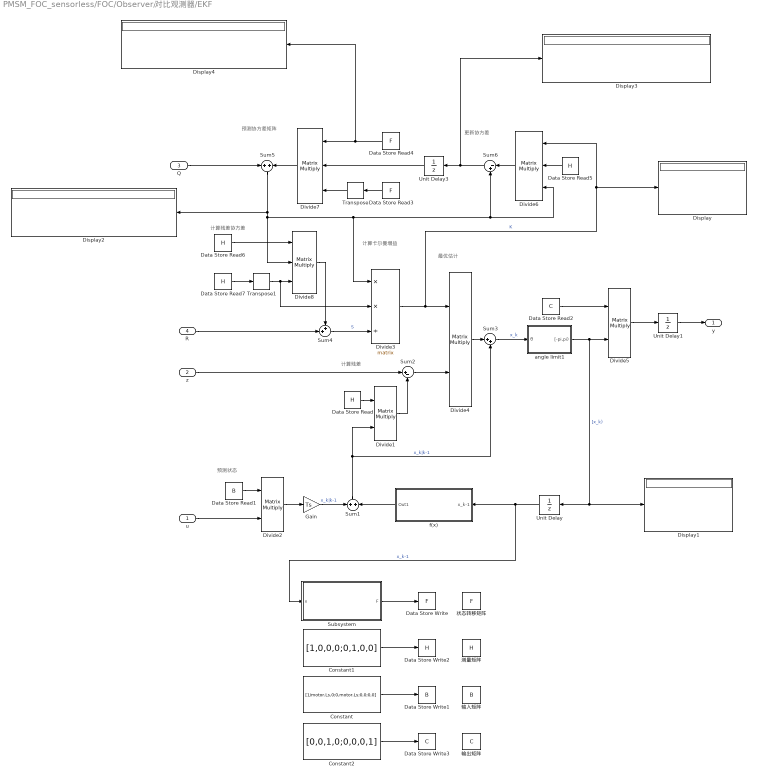
== system PMSM_FOC_sensorless/FOC/Observer/对比观测器/EKF ==
  note: 预测状态
  note: 计算残差
  note: 最优估计
  note: 计算残差协方差
  note: 预测协方差矩阵
  note: 计算卡尔曼增益
  note: 更新协方差
  u : Inport
  z : Inport  Port=2
  Q : Inport  Port=3
  R : Inport  Port=4
  Constant : Constant  Value=[1/motor.Ls,0;0,motor.Ls;0,0;0,0]  VectorParams1D=off  OutDataTypeStr=single
  Constant1 : Constant  Value=[1,0,0,0;0,1,0,0]  VectorParams1D=off  OutDataTypeStr=single
  Constant2 : Constant  Value=[0,0,1,0;0,0,0,1]  VectorParams1D=off  OutDataTypeStr=single
  Data Store Read{,5..7} (4 alike) : DataStoreRead  DataStoreName=H  IndexOptions=Index vector (dialog)  Indices=1  OutputSizes=1
  Data Store Read1 : DataStoreRead  DataStoreName=B  IndexOptions=Index vector (dialog)  Indices=1  OutputSizes=1
  Data Store Read2 : DataStoreRead  DataStoreName=C  IndexOptions=Index vector (dialog)  Indices=1  OutputSizes=1
  Data Store Read3 : DataStoreRead  DataStoreName=F  IndexOptions=Index vector (dialog)  Indices=1  OutputSizes=1
  Data Store Read4 : DataStoreRead  DataStoreName=F  IndexOptions=Index vector (dialog)  Indices=1  OutputSizes=1
  Data Store Write : DataStoreWrite  DataStoreName=F  IndexOptions=Index vector (dialog)  Indices=1  OutputSizes=1
  Data Store Write1 : DataStoreWrite  DataStoreName=B  IndexOptions=Index vector (dialog)  Indices=1  OutputSizes=1
  Data Store Write2 : DataStoreWrite  DataStoreName=H  IndexOptions=Index vector (dialog)  Indices=1  OutputSizes=1
  Data Store Write3 : DataStoreWrite  DataStoreName=C  IndexOptions=Index vector (dialog)  Indices=1  OutputSizes=1
  Display{,1..4} (5 alike) : Display
  Divide{1..2,4..5} (4 alike) : Product  Inputs=**  Multiplication=Matrix(*)
  Divide3 : Product  Inputs=**/  Multiplication=Matrix(*)
  Divide6 : Product  Inputs=***  Multiplication=Matrix(*)
  Divide7 : Product  Inputs=***  Multiplication=Matrix(*)
  Divide8 : Product  Inputs=***  Multiplication=Matrix(*)
  Gain : Gain  Gain=Ts
  Subsystem : Subsystem
  Sum1 : Sum  Inputs=+|+
  Sum2 : Sum  Inputs=|+-
  Sum3 : Sum  Inputs=|++
  Sum4 : Sum  Inputs=++|
  Sum5 : Sum  Inputs=+|+
  Sum6 : Sum  Inputs=|-+
  Transpose : matrix_library/Transpose
  Transpose1 : matrix_library/Transpose
  Unit Delay : UnitDelay  InitialCondition=zeros(4,1)  SampleTime=-1
  Unit Delay1 : UnitDelay  InitialCondition=zeros(2,1)  SampleTime=-1
  Unit Delay3 : UnitDelay  InitialCondition=diag([1e0,1e0,1000*[1,Ts^2/4]])  SampleTime=-1
  angle limit1 : Subsystem
  f(x) : Subsystem
  测量矩阵 : DataStoreMemory  DataStoreName=H  WriteAfterWriteMsg=warning  InitialValue=[1,0,0,0;0,1,0,0]  VectorParams1D=off  ShowAdditionalParam=off
  状态转移矩阵 : DataStoreMemory  DataStoreName=F  WriteAfterWriteMsg=warning  InitialValue=eye(4)  VectorParams1D=off  ShowAdditionalParam=off
  输入矩阵 : DataStoreMemory  DataStoreName=B  WriteAfterWriteMsg=warning  InitialValue=[1/motor.Ls,0;0,motor.Ls;0,0;0,0]  VectorParams1D=off  ShowAdditionalParam=off
  输出矩阵 : DataStoreMemory  DataStoreName=C  WriteAfterWriteMsg=warning  InitialValue=[0,0,1,0;0,0,0,1]  VectorParams1D=off  ShowAdditionalParam=off
  y : Outport
  wires:
  Sum3/1 -> angle limit1/1(θ)  "x_k"
  Divide3/1 -> Display/1, Divide6/1, Divide4/1  "K"
  Sum1/1 -> Divide1/2, Sum3/2  "x_k|k-1"
  u/1 -> Divide2/2
  Data Store Read2/1 -> Divide5/1
  Unit Delay/1 -> Subsystem/1(x), f(x)/1(x_k-1)  "x_k-1"
  Divide2/1 -> Gain/1
  Divide4/1 -> Sum3/1
  Sum2/1 -> Divide4/2
  z/1 -> Sum2/1
  Data Store Read1/1 -> Divide2/1
  Divide5/1 -> Unit Delay1/1
  Constant/1 -> Data Store Write1/1
  Constant1/1 -> Data Store Write2/1
  Q/1 -> Sum5/1
  Sum5/1 -> Divide3/1, Divide6/3, Sum6/2, Divide8/2, Display2/1
  Divide7/1 -> Sum5/2
  R/1 -> Sum4/2
  Unit Delay3/1 -> Divide7/2
  Sum4/1 -> Divide3/3  "S"
  Data Store Read3/1 -> Transpose/1
  Data Store Read5/1 -> Divide6/2
  Divide6/1 -> Sum6/1
  Transpose/1 -> Divide7/3
  Subsystem/1(F) -> Data Store Write/1
  f(x)/1(Out1) -> Sum1/2
  angle limit1/1("[-pi,pi)") -> Divide5/2, Display1/1, Unit Delay/1  "[x_k)"
  Gain/1 -> Sum1/1  "x_k|k-1"
  Data Store Read/1 -> Divide1/1
  Divide1/1 -> Sum2/2
  Constant2/1 -> Data Store Write3/1
  Data Store Read7/1 -> Transpose1/1
  Transpose1/1 -> Divide3/2, Divide8/3
  Data Store Read6/1 -> Divide8/1
  Divide8/1 -> Sum4/1
  Unit Delay1/1 -> y/1
  Sum6/1 -> Display3/1, Unit Delay3/1
  Data Store Read4/1 -> Display4/1, Divide7/1

== system PMSM_FOC_sensorless/FOC/Observer/对比观测器/FKF ==
  z : Inport
  u : Inport  Port=2
  AKF : Subsystem
  Demux : Demux  Outputs=2
  位置提取 : Subsystem
  角度转换 : Subsystem
  计算转子反电动势 : Subsystem
  转矩计算 : Subsystem
  ω_m : Outport
  θ_e : Outport  Port=2
  wires:
  转矩计算/1(T) -> AKF/1(u_k)  "T"
  z/1 -> 计算转子反电动势/1(Iαβ), 转矩计算/2(I_αβ)
  计算转子反电动势/1(Eαβ) -> 位置提取/1(Eαβ)  "E_αβ"
  Demux/2 -> θ_e/1, 角度转换/1(θ)
  Demux/1 -> ω_m/1
  u/1 -> 计算转子反电动势/2(Uαβ)
  AKF/1(x_k) -> Demux/1
  角度转换/1(sincos) -> 转矩计算/1(θ_sincos), 位置提取/2(θ_sincos)
  位置提取/1(ωθ) -> AKF/2(z_k)  "ωθ~"

== system PMSM_FOC_sensorless/FOC/Observer/对比观测器/Subsystem ==
  θ_e : Inport
  Constant2 : Constant  Value=-pi  OutDataTypeStr=single
  Constant4 : Constant  Value=pi  OutDataTypeStr=single
  Difference : simulink/Discrete/Difference  ICPrevInput=0.0  OutMin=[]  OutMax=[]  OutDataType=fixdt(1, 16)  OutScaling=2^-10  DoSatur=off
  Gain : Gain  Gain=1/(motor.P*Ts)
  Gain6 : Gain  Gain=-2*pi  OutDataTypeStr=single
  Gain7 : Gain  Gain=2*pi  OutDataTypeStr=single
  Relational Operator2 : RelationalOperator  Operator=<  RndMeth=Simplest  InputSameDT=off
  Relational Operator3 : RelationalOperator  Operator=<=  RndMeth=Simplest  InputSameDT=off
  Sum3 : Sum  Inputs=+++
  Y : Outport
  wires:
  θ_e/1 -> Difference/1
  Sum3/1 -> Gain/1
  Difference/1 -> Relational Operator2/1, Sum3/2, Relational Operator3/2
  Gain6/1 -> Sum3/1
  Relational Operator2/1 -> Gain7/1
  Constant4/1 -> Relational Operator3/1
  Gain7/1 -> Sum3/3
  Relational Operator3/1 -> Gain6/1
  Constant2/1 -> Relational Operator2/2
  Gain/1 -> Y/1

== system PMSM_FOC_sensorless/FOC/Observer/对比观测器/Subsystem1 ==
  0-2pi : Inport
  Constant3 : Constant  Value=-pi  OutDataTypeStr=single
  Constant4 : Constant  Value=pi  OutDataTypeStr=single
  Gain6 : Gain  Gain=-2*pi  OutDataTypeStr=single
  Gain7 : Gain  Gain=2*pi  OutDataTypeStr=single
  Relational Operator2 : RelationalOperator  Operator=<  RndMeth=Simplest  InputSameDT=off
  Relational Operator3 : RelationalOperator  Operator=<  RndMeth=Simplest  InputSameDT=off
  Sum3 : Sum  Inputs=+++
  -pi-pi : Outport
  wires:
  Constant4/1 -> Relational Operator3/1
  Constant3/1 -> Relational Operator2/2
  0-2pi/1 -> Relational Operator2/1, Sum3/2, Relational Operator3/2
  Relational Operator2/1 -> Gain7/1
  Relational Operator3/1 -> Gain6/1
  Gain6/1 -> Sum3/1
  Gain7/1 -> Sum3/3
  Sum3/1 -> -pi-pi/1

== system PMSM_FOC_sensorless/FOC/Observer/对比观测器/Subsystem2 ==
  0-2pi : Inport
  Constant3 : Constant  Value=-pi  OutDataTypeStr=single
  Constant4 : Constant  Value=pi  OutDataTypeStr=single
  Gain6 : Gain  Gain=-2*pi  OutDataTypeStr=single
  Gain7 : Gain  Gain=2*pi  OutDataTypeStr=single
  Relational Operator2 : RelationalOperator  Operator=<  RndMeth=Simplest  InputSameDT=off
  Relational Operator3 : RelationalOperator  Operator=<  RndMeth=Simplest  InputSameDT=off
  Sum3 : Sum  Inputs=+++
  -pi-pi : Outport
  wires:
  Sum3/1 -> -pi-pi/1
  Gain7/1 -> Sum3/3
  Gain6/1 -> Sum3/1
  Relational Operator3/1 -> Gain6/1
  Relational Operator2/1 -> Gain7/1
  0-2pi/1 -> Relational Operator3/2, Sum3/2, Relational Operator2/1
  Constant3/1 -> Relational Operator2/2
  Constant4/1 -> Relational Operator3/1

== system PMSM_FOC_sensorless/FOC/Observer/对比观测器/Subsystem3 ==
  0-2pi : Inport
  Constant3 : Constant  Value=-pi  OutDataTypeStr=single
  Constant4 : Constant  Value=pi  OutDataTypeStr=single
  Gain6 : Gain  Gain=-2*pi  OutDataTypeStr=single
  Gain7 : Gain  Gain=2*pi  OutDataTypeStr=single
  Relational Operator2 : RelationalOperator  Operator=<  RndMeth=Simplest  InputSameDT=off
  Relational Operator3 : RelationalOperator  Operator=<  RndMeth=Simplest  InputSameDT=off
  Sum3 : Sum  Inputs=+++
  -pi-pi : Outport
  wires:
  Constant4/1 -> Relational Operator3/1
  Constant3/1 -> Relational Operator2/2
  0-2pi/1 -> Relational Operator2/1, Sum3/2, Relational Operator3/2
  Relational Operator2/1 -> Gain7/1
  Relational Operator3/1 -> Gain6/1
  Gain6/1 -> Sum3/1
  Gain7/1 -> Sum3/3
  Sum3/1 -> -pi-pi/1

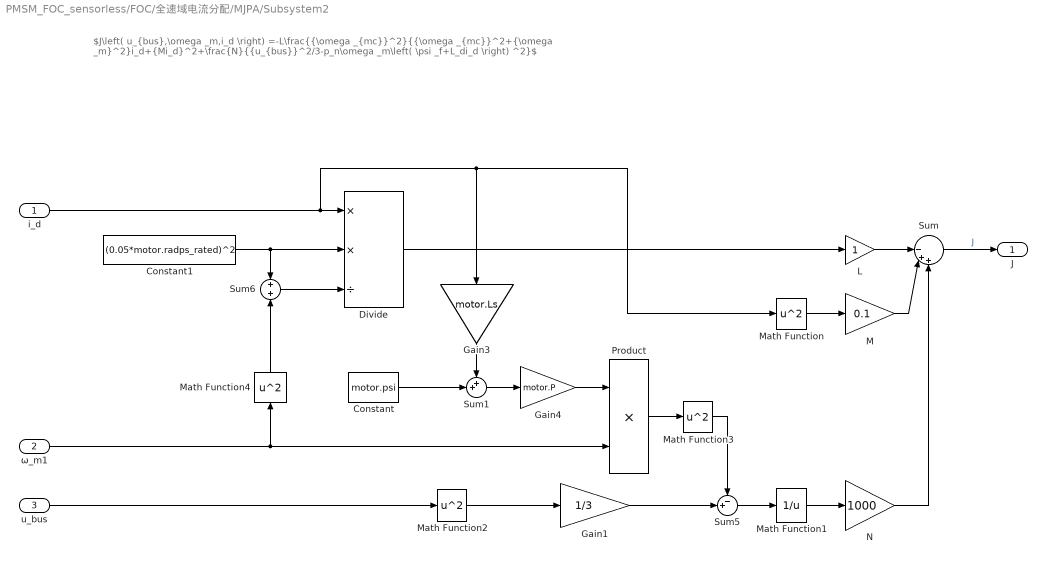
== system PMSM_FOC_sensorless/FOC/全速域电流分配/MJPA/Subsystem2 ==
  note: $J\left( u_{bus},\omega _m,i_d \right) =-L\frac{{\omega _{mc}}^2}{{\omega _{mc}}^2+{\omega _m}^2}i_d+{Mi_d}^2+\frac{N}{{u_{bus}}^2/3-p_n\omega _m\left( \psi _f+L_di_d \right) ^2}$
  i_d : Inport
  ω_m1 : Inport  Port=2
  u_bus : Inport  Port=3
  Constant : Constant  Value=motor.psi  OutDataTypeStr=single
  Constant1 : Constant  Value=(0.05*motor.radps_rated)^2  OutDataTypeStr=single
  Divide : Product  Inputs=**/
  Gain1 : Gain  Gain=1/3
  Gain3 : Gain  Gain=motor.Ls
  Gain4 : Gain  Gain=motor.P
  L : Gain
  M : Gain  Gain=0.1
  Math Function{,2..4} (4 alike) : Math  Operator=square
  Math Function1 : Math  Operator=reciprocal
  N : Gain  Gain=1000
  Product : Product
  Sum : Sum  Inputs=||-++
  Sum1 : Sum  Inputs=++|
  Sum5 : Sum  Inputs=-+|
  Sum6 : Sum  Inputs=+|+
  J : Outport
  wires:
  Divide/1 -> L/1
  Gain3/1 -> Sum1/1
  Sum1/1 -> Gain4/1
  u_bus/1 -> Math Function2/1
  Sum5/1 -> Math Function1/1
  L/1 -> Sum/1
  Constant/1 -> Sum1/2
  Math Function4/1 -> Sum6/2
  Math Function/1 -> M/1
  M/1 -> Sum/2
  i_d/1 -> Math Function/1, Gain3/1, Divide/1
  Sum6/1 -> Divide/3
  ω_m1/1 -> Math Function4/1, Product/2
  N/1 -> Sum/3
  Math Function1/1 -> N/1
  Gain1/1 -> Sum5/2
  Product/1 -> Math Function3/1
  Sum/1 -> J/1  "J"
  Constant1/1 -> Sum6/1, Divide/2
  Math Function2/1 -> Gain1/1
  Math Function3/1 -> Sum5/1
  Gain4/1 -> Product/1

== system PMSM_FOC_sensorless/FOC/Observer/AKF/协方差估计/乘法积分器 ==
  note: 矩阵指数运算量比较大，用一阶泰勒展开式近似
  S~ : Inport
  S : Inport  Port=2
  Divide1 : Product  Inputs=*/  Multiplication=Matrix(*)
  Divide2 : Product  Inputs=***  Multiplication=Matrix(*)
  Gain1 : Gain  Gain=FAKF.fg
  Gain2 : Gain  Gain=1-FAKF.fg
  Sum3 : Sum  Inputs=|++
  Transpose2 : matrix_library/Transpose
  Unit Delay2 : UnitDelay  InitialCondition=eye(2)  SampleTime=-1
  Q : Outport
  wires:
  Unit Delay2/1 -> Divide2/2, Gain2/1
  Divide2/1 -> Gain1/1
  Gain2/1 -> Sum3/2
  Divide1/1 -> Divide2/1, Transpose2/1
  Gain1/1 -> Sum3/1
  Transpose2/1 -> Divide2/3
  Sum3/1 -> Unit Delay2/1, Q/1
  S~/1 -> Divide1/1
  S/1 -> Divide1/2

== system PMSM_FOC_sensorless/FOC/Observer/AKF/协方差估计/乘法积分器1 ==
  note: 矩阵指数运算量比较大，用一阶泰勒展开式近似
  T~ : Inport
  T : Inport  Port=2
  Divide1 : Product  Inputs=*/  Multiplication=Matrix(*)
  Divide2 : Product  Inputs=***  Multiplication=Matrix(*)
  Gain1 : Gain  Gain=FAKF.fg
  Gain2 : Gain  Gain=1-FAKF.fg
  Sum3 : Sum  Inputs=|++
  Transpose2 : matrix_library/Transpose
  Unit Delay2 : UnitDelay  InitialCondition=eye(2)  SampleTime=-1
  R : Outport
  wires:
  T/1 -> Divide1/2
  T~/1 -> Divide1/1
  Sum3/1 -> R/1, Unit Delay2/1
  Transpose2/1 -> Divide2/3
  Gain1/1 -> Sum3/1
  Divide1/1 -> Transpose2/1, Divide2/1
  Gain2/1 -> Sum3/2
  Divide2/1 -> Gain1/1
  Unit Delay2/1 -> Gain2/1, Divide2/2

== system PMSM_FOC_sensorless/FOC/Observer/AKF/协方差估计/息差估计 ==
  ωθ : Inport
  Demux1 : Demux  Outputs=2
  IIR Filter1 : mcbcontrolslib/IIR Filter  VariantControl=Low Pass Filter  VariantSelect=Low-pass  FilterConstantInputType=Specify via dialog  Filter_constant=FAKF.fg  InitialOutput=Specify via dialog  InitialOutputValue=0  ExternalReset=none  advancedSettings=off  Ts=50e-6  cutOff_freq=167.5315
  Matrix Concatenate : Concatenate  Mode=Multidimensional array
  Matrix Concatenate1 : Concatenate  Mode=Multidimensional array
  Matrix Concatenate2 : Concatenate  Mode=Multidimensional array  ConcatenateDimension=2
  Product : Product
  Product1 : Product
  Product3 : Product
  cov : Outport
  wires:
  Demux1/1 -> Product1/1, Product/1, Product/2
  Matrix Concatenate2/1 -> IIR Filter1/1
  Matrix Concatenate1/1 -> Matrix Concatenate2/2
  Matrix Concatenate/1 -> Matrix Concatenate2/1
  Product/1 -> Matrix Concatenate/1
  Product1/1 -> Matrix Concatenate/2, Matrix Concatenate1/1
  Product3/1 -> Matrix Concatenate1/2
  ωθ/1 -> Demux1/1
  Demux1/2 -> Product3/2, Product3/1, Product1/2
  IIR Filter1/1 -> cov/1

== system PMSM_FOC_sensorless/FOC/Observer/AKF/协方差估计/残差估计 ==
  ωθ : Inport
  Demux1 : Demux  Outputs=2
  Gain : Gain  Gain=Ts/2
  IIR Filter1 : mcbcontrolslib/IIR Filter  VariantControl=Low Pass Filter  VariantSelect=Low-pass  FilterConstantInputType=Specify via dialog  Filter_constant=FAKF.fg  InitialOutput=Specify via dialog  InitialOutputValue=0  ExternalReset=none  advancedSettings=off  Ts=50e-6  cutOff_freq=167.5315
  Matrix Concatenate : Concatenate  Mode=Multidimensional array
  Matrix Concatenate1 : Concatenate  Mode=Multidimensional array
  Matrix Concatenate2 : Concatenate  Mode=Multidimensional array  ConcatenateDimension=2
  Product : Product
  Product1 : Product
  Product3 : Product
  cov : Outport
  wires:
  Gain/1 -> Product1/2, Product3/2, Product3/1
  ωθ/1 -> Demux1/1
  Product3/1 -> Matrix Concatenate1/2
  Product1/1 -> Matrix Concatenate1/1, Matrix Concatenate/2
  Product/1 -> Matrix Concatenate/1
  Matrix Concatenate/1 -> Matrix Concatenate2/1
  Matrix Concatenate1/1 -> Matrix Concatenate2/2
  Matrix Concatenate2/1 -> IIR Filter1/1
  IIR Filter1/1 -> cov/1
  Demux1/1 -> Gain/1, Product/2, Product/1, Product1/1

== system PMSM_FOC_sensorless/FOC/Observer/AKF/状态观测/angle limit1 ==
  In : Inport
  Constant2 : Constant  Value=-pi  OutDataTypeStr=single
  Constant4 : Constant  Value=pi  OutDataTypeStr=single
  Demux : Demux  Outputs=2
  Gain6 : Gain  Gain=-2*pi  OutDataTypeStr=single
  Gain7 : Gain  Gain=2*pi  OutDataTypeStr=single
  Mux : Mux  Inputs=2
  Relational Operator2 : RelationalOperator  Operator=<  RndMeth=Simplest  InputSameDT=off
  Relational Operator3 : RelationalOperator  Operator=<  RndMeth=Simplest  InputSameDT=off
  Sum3 : Sum  Inputs=+++
  P_k1 : Outport
  wires:
  Demux/1 -> Mux/1
  Mux/1 -> P_k1/1
  In/1 -> Demux/1
  Sum3/1 -> Mux/2
  Gain6/1 -> Sum3/1
  Relational Operator2/1 -> Gain7/1
  Gain7/1 -> Sum3/3
  Relational Operator3/1 -> Gain6/1
  Constant4/1 -> Relational Operator3/1
  Demux/2 -> Relational Operator2/1, Sum3/2, Relational Operator3/2
  Constant2/1 -> Relational Operator2/2

== system PMSM_FOC_sensorless/FOC/Observer/AKF/状态观测/angle limit2 ==
  In : Inport
  Constant2 : Constant  Value=-pi  OutDataTypeStr=single
  Constant4 : Constant  Value=pi  OutDataTypeStr=single
  Demux : Demux  Outputs=2
  Gain6 : Gain  Gain=-2*pi  OutDataTypeStr=single
  Gain7 : Gain  Gain=2*pi  OutDataTypeStr=single
  Mux : Mux  Inputs=2
  Relational Operator2 : RelationalOperator  Operator=<  RndMeth=Simplest  InputSameDT=off
  Relational Operator3 : RelationalOperator  Operator=<  RndMeth=Simplest  InputSameDT=off
  Sum3 : Sum  Inputs=+++
  P_k1 : Outport
  wires:
  Demux/1 -> Mux/1
  Mux/1 -> P_k1/1
  In/1 -> Demux/1
  Sum3/1 -> Mux/2
  Gain6/1 -> Sum3/1
  Relational Operator2/1 -> Gain7/1
  Gain7/1 -> Sum3/3
  Relational Operator3/1 -> Gain6/1
  Constant4/1 -> Relational Operator3/1
  Demux/2 -> Relational Operator2/1, Sum3/2, Relational Operator3/2
  Constant2/1 -> Relational Operator2/2

== system PMSM_FOC_sensorless/FOC/Observer/AKF/状态观测/angle limit3 ==
  In : Inport
  Constant2 : Constant  Value=-pi  OutDataTypeStr=single
  Constant4 : Constant  Value=pi  OutDataTypeStr=single
  Demux : Demux  Outputs=2
  Gain6 : Gain  Gain=-2*pi  OutDataTypeStr=single
  Gain7 : Gain  Gain=2*pi  OutDataTypeStr=single
  Mux : Mux  Inputs=2
  Relational Operator2 : RelationalOperator  Operator=<  RndMeth=Simplest  InputSameDT=off
  Relational Operator3 : RelationalOperator  Operator=<  RndMeth=Simplest  InputSameDT=off
  Sum3 : Sum  Inputs=+++
  x : Outport
  wires:
  Constant2/1 -> Relational Operator2/2
  Demux/2 -> Relational Operator3/2, Sum3/2, Relational Operator2/1
  Constant4/1 -> Relational Operator3/1
  Relational Operator3/1 -> Gain6/1
  Gain7/1 -> Sum3/3
  Relational Operator2/1 -> Gain7/1
  Gain6/1 -> Sum3/1
  Sum3/1 -> Mux/2
  In/1 -> Demux/1
  Mux/1 -> x/1
  Demux/1 -> Mux/1

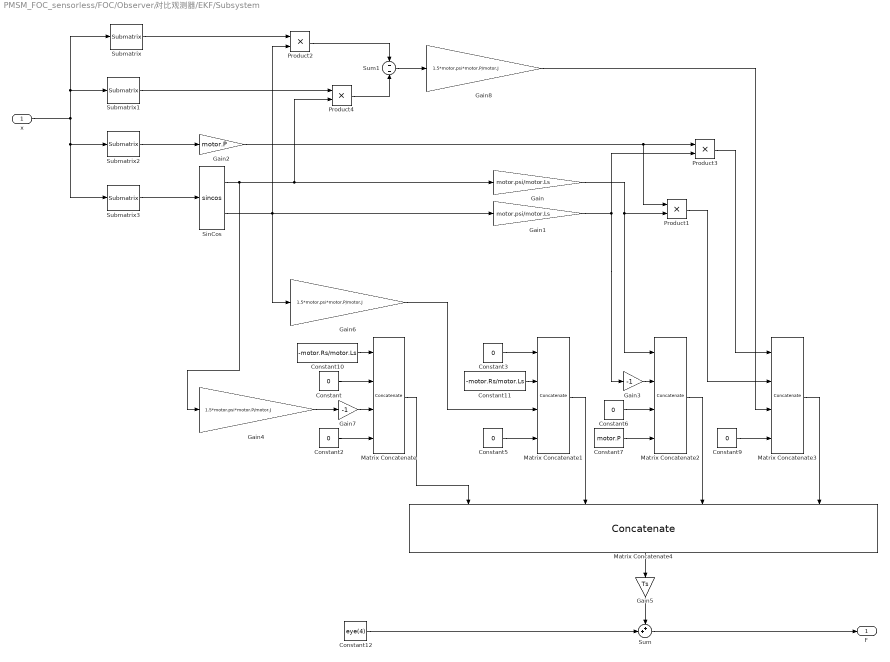
== system PMSM_FOC_sensorless/FOC/Observer/对比观测器/EKF/Subsystem ==
  x : Inport
  Constant{,2..3,5..6,9} (6 alike) : Constant  Value=0  OutDataTypeStr=single
  Constant10 : Constant  Value=-motor.Rs/motor.Ls  OutDataTypeStr=single
  Constant11 : Constant  Value=-motor.Rs/motor.Ls  OutDataTypeStr=single
  Constant12 : Constant  Value=eye(4)  OutDataTypeStr=single
  Constant7 : Constant  Value=motor.P  OutDataTypeStr=single
  Gain : Gain  Gain=motor.psi/motor.Ls
  Gain1 : Gain  Gain=motor.psi/motor.Ls
  Gain2 : Gain  Gain=motor.P
  Gain3 : Gain  Gain=-1
  Gain4 : Gain  Gain=1.5*motor.psi*motor.P/motor.J
  Gain5 : Gain  Gain=Ts
  Gain6 : Gain  Gain=1.5*motor.psi*motor.P/motor.J
  Gain7 : Gain  Gain=-1
  Gain8 : Gain  Gain=1.5*motor.psi*motor.P/motor.J
  Matrix Concatenate{,1..3} (4 alike) : Concatenate  NumInputs=4  Mode=Multidimensional array
  Matrix Concatenate4 : Concatenate  NumInputs=4  Mode=Multidimensional array  ConcatenateDimension=2
  Product{1..4} (4 alike) : Product
  SinCos : Trigonometry  Operator=sincos
  Submatrix : matrix_library/Submatrix  RowSpan=Range of rows  RowStartMode=Index  RowStartIndex=1  RowEndMode=Index  RowEndIndex=1  ColSpan=One column  ColStartMode=First  ColStartIndex=1  ColEndMode=Index  ColEndIndex=1
  Submatrix1 : matrix_library/Submatrix  RowSpan=Range of rows  RowStartMode=Index  RowStartIndex=2  RowEndMode=Index  RowEndIndex=2  ColSpan=One column  ColStartMode=First  ColStartIndex=1  ColEndMode=Index  ColEndIndex=1
  Submatrix2 : matrix_library/Submatrix  RowSpan=Range of rows  RowStartMode=Index  RowStartIndex=3  RowEndMode=Index  RowEndIndex=3  ColSpan=One column  ColStartMode=First  ColStartIndex=1  ColEndMode=Index  ColEndIndex=1
  Submatrix3 : matrix_library/Submatrix  RowSpan=Range of rows  RowStartMode=Index  RowStartIndex=4  RowEndMode=Index  RowEndIndex=4  ColSpan=One column  ColStartMode=First  ColStartIndex=1  ColEndMode=Index  ColEndIndex=1
  Sum : Sum  Inputs=++|
  Sum1 : Sum  Inputs=-|-
  F : Outport
  wires:
  Constant2/1 -> Matrix Concatenate/4
  Constant/1 -> Matrix Concatenate/2
  Constant3/1 -> Matrix Concatenate1/1
  Constant5/1 -> Matrix Concatenate1/4
  Matrix Concatenate/1 -> Matrix Concatenate4/1
  Constant7/1 -> Matrix Concatenate2/4
  Sum/1 -> F/1
  Constant6/1 -> Matrix Concatenate2/3
  Constant10/1 -> Matrix Concatenate/1
  Gain8/1 -> Matrix Concatenate3/3
  Gain6/1 -> Matrix Concatenate1/3
  Matrix Concatenate1/1 -> Matrix Concatenate4/2
  Gain4/1 -> Gain7/1
  Matrix Concatenate2/1 -> Matrix Concatenate4/3
  Constant11/1 -> Matrix Concatenate1/2
  Constant9/1 -> Matrix Concatenate3/4
  Matrix Concatenate3/1 -> Matrix Concatenate4/4
  Gain/1 -> Matrix Concatenate2/1, Product1/2
  Product3/1 -> Matrix Concatenate3/1
  Product1/1 -> Matrix Concatenate3/2
  x/1 -> Submatrix3/1, Submatrix2/1, Submatrix1/1, Submatrix/1
  SinCos/1 -> Gain/1, Product4/2, Gain4/1
  SinCos/2 -> Gain6/1, Product2/2, Gain1/1
  Gain1/1 -> Product3/2, Gain3/1
  Constant12/1 -> Sum/2
  Matrix Concatenate4/1 -> Gain5/1
  Gain5/1 -> Sum/1
  Submatrix3/1 -> SinCos/1
  Submatrix2/1 -> Gain2/1
  Gain2/1 -> Product1/1, Product3/1
  Gain3/1 -> Matrix Concatenate2/2
  Gain7/1 -> Matrix Concatenate/3
  Submatrix/1 -> Product2/1
  Submatrix1/1 -> Product4/1
  Product2/1 -> Sum1/1
  Product4/1 -> Sum1/2
  Sum1/1 -> Gain8/1
